simulink model "problem5"  (R2020a)
settings: Solver=VariableStepAuto  StartTime=0.0  StopTime=10.0  RelTol=1e-3
model workspace (MAT data in the model file):
  C = 10
  R = 10
settings Model: Creator=kasutav  LastModifiedBy=kasutav

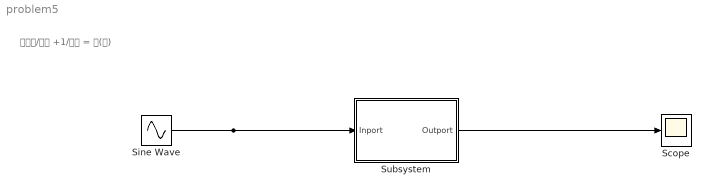
== system problem5 ==
  note: 𝑅𝑑𝑄/𝑑𝑡 +1/𝐶𝑄 = 𝐸(𝑡)
  Scope : Scope
  Sine Wave : Sin  Amplitude=50  SampleTime=0
  Subsystem : Subsystem
  wires:
  Sine Wave/1 -> Subsystem/1(Inport)
  Subsystem/1(Outport) -> Scope/1

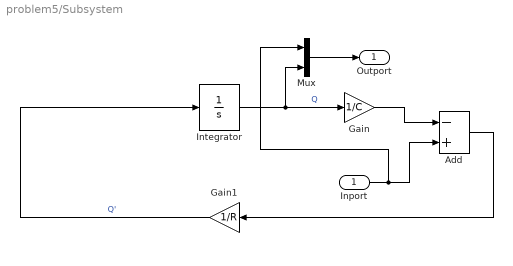
== system problem5/Subsystem ==
  Inport : Inport
  Add : Sum  Inputs=-+
  Gain : Gain  Gain=1/C
  Gain1 : Gain  Gain=1/R
  Integrator : Integrator  InitialCondition=4
  Mux : Mux  Inputs=2
  Outport : Outport
  wires:
  Add/1 -> Gain1/1
  Mux/1 -> Outport/1
  Inport/1 -> Mux/1, Add/2
  Gain1/1 -> Integrator/1  "Q'"
  Gain/1 -> Add/1
  Integrator/1 -> Mux/2, Gain/1  "Q"
